simulink model "logic"  (R2023a)
settings: Solver=FixedStepAuto  StartTime=0.0  StopTime=10.0  FixedStep=1  RelTol=1e-3
libraries: simulink x1
settings Model: Creator=Dheeraj Patil  LastModifiedBy=Dheeraj Patil

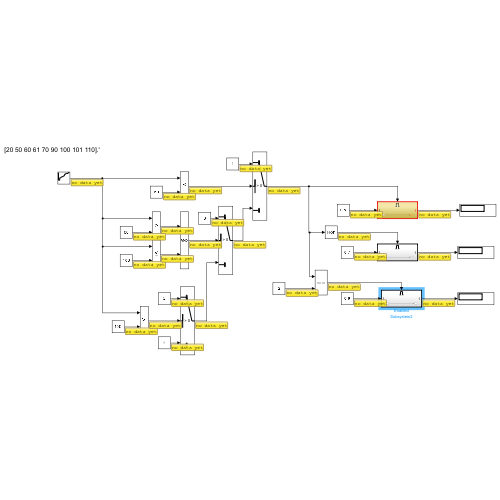
[thumbnail: Simulink's stored preview of the top-level diagram]
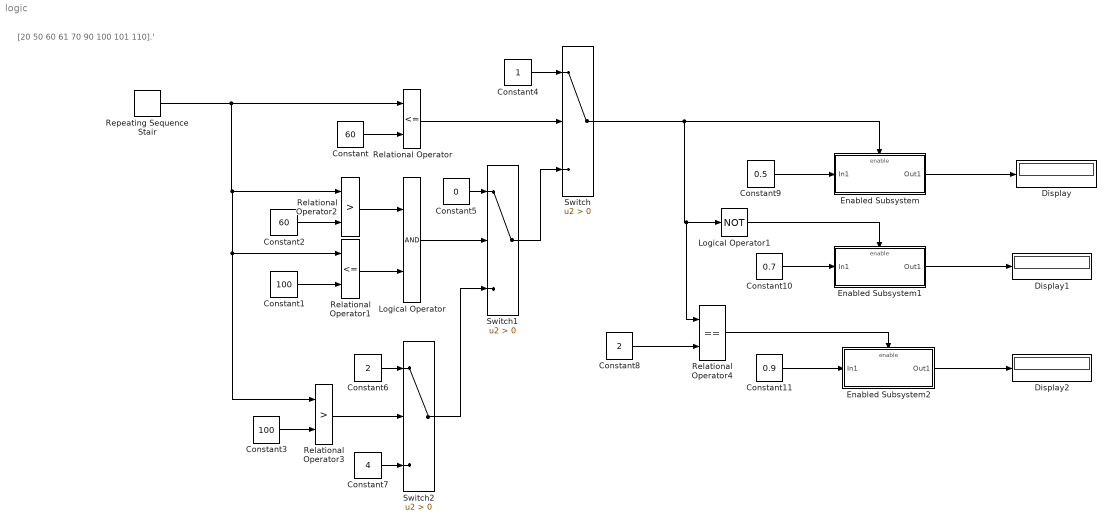
== system logic ==
  note: [20 50 60 61 70 90 100 101 110].'
  Constant : Constant  Value=60
  Constant1 : Constant  Value=100
  Constant10 : Constant  Value=0.7
  Constant11 : Constant  Value=0.9
  Constant2 : Constant  Value=60
  Constant3 : Constant  Value=100
  Constant4 : Constant
  Constant5 : Constant  Value=0
  Constant6 : Constant  Value=2
  Constant7 : Constant  Value=4
  Constant8 : Constant  Value=2
  Constant9 : Constant  Value=0.5
  Display : Display
  Display1 : Display
  Display2 : Display
  Enabled Subsystem : Subsystem  TreatAsAtomicUnit=on
      settings: LibrarySourceBlock=|
      | hdlsllib/Ports &
      | Subsystems/Enabled
      | Subsystem
  Enabled Subsystem1 : Subsystem  TreatAsAtomicUnit=on
      settings: LibrarySourceBlock=|
      | hdlsllib/Ports &
      | Subsystems/Enabled
      | Subsystem
  Enabled Subsystem2 : Subsystem  TreatAsAtomicUnit=on
      settings: LibrarySourceBlock=|
      | hdlsllib/Ports &
      | Subsystems/Enabled
      | Subsystem
  Logical Operator : Logic  AllPortsSameDT=off  OutDataTypeStr=boolean
  Logical Operator1 : Logic  Operator=NOT  AllPortsSameDT=off  OutDataTypeStr=boolean
  Relational Operator : RelationalOperator  Operator=<=  OutDataTypeStr=boolean  RndMeth=Simplest  InputSameDT=off
  Relational Operator1 : RelationalOperator  Operator=<=  OutDataTypeStr=boolean  RndMeth=Simplest  InputSameDT=off
  Relational Operator2 : RelationalOperator  Operator=>  OutDataTypeStr=boolean  RndMeth=Simplest  InputSameDT=off
  Relational Operator3 : RelationalOperator  Operator=>  OutDataTypeStr=boolean  RndMeth=Simplest  InputSameDT=off
  Relational Operator4 : RelationalOperator  Operator===  OutDataTypeStr=boolean  RndMeth=Simplest  InputSameDT=off
  Repeating Sequence Stair : simulink/Sources/Repeating Sequence Stair  OutValues=[20 50 60 61 70 90 100 101 110].'  tsamp=-1  OutMin=[]  OutMax=[]  OutDataTypeStr=double  OutputDataTypeScalingMode=double  OutDataType=fixdt(0,8)  ConRadixGroup=Best Precision: Vector-wise  OutScaling=2^-12
  Switch : Switch  Criteria=u2 > Threshold  SaturateOnIntegerOverflow=off  InputSameDT=off
  Switch1 : Switch  Criteria=u2 > Threshold  SaturateOnIntegerOverflow=off  InputSameDT=off
  Switch2 : Switch  Criteria=u2 > Threshold  SaturateOnIntegerOverflow=off  InputSameDT=off
  wires:
  Relational Operator/1 -> Switch/2
  Constant/1 -> Relational Operator/2
  Switch1/1 -> Switch/3
  Constant1/1 -> Relational Operator1/2
  Logical Operator/1 -> Switch1/2
  Relational Operator1/1 -> Logical Operator/2
  Relational Operator2/1 -> Logical Operator/1
  Constant2/1 -> Relational Operator2/2
  Repeating Sequence Stair/1 -> Relational Operator1/1, Relational Operator3/1, Relational Operator2/1, Relational Operator/1
  Switch2/1 -> Switch1/3
  Relational Operator3/1 -> Switch2/2
  Constant3/1 -> Relational Operator3/2
  Constant4/1 -> Switch/1
  Constant5/1 -> Switch1/1
  Constant6/1 -> Switch2/1
  Constant7/1 -> Switch2/3
  Switch/1 -> Relational Operator4/1, Logical Operator1/1, Enabled Subsystem/Enable
  Logical Operator1/1 -> Enabled Subsystem1/Enable
  Constant8/1 -> Relational Operator4/2
  Relational Operator4/1 -> Enabled Subsystem2/Enable
  Enabled Subsystem/1(Out1) -> Display/1
  Constant9/1 -> Enabled Subsystem/1(In1)
  Constant10/1 -> Enabled Subsystem1/1(In1)
  Enabled Subsystem1/1(Out1) -> Display1/1
  Constant11/1 -> Enabled Subsystem2/1(In1)
  Enabled Subsystem2/1(Out1) -> Display2/1

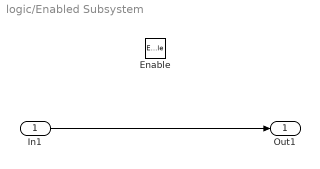
== system logic/Enabled Subsystem ==
  In1 : Inport
  Enable : EnablePort
  Out1 : Outport  OutputWhenDisabled=reset  InitialOutput=0
  wires:
  In1/1 -> Out1/1

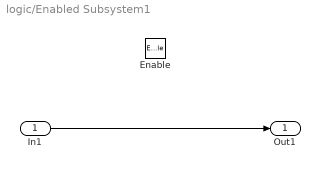
== system logic/Enabled Subsystem1 ==
  In1 : Inport
  Enable : EnablePort
  Out1 : Outport  OutputWhenDisabled=reset  InitialOutput=0
  wires:
  In1/1 -> Out1/1

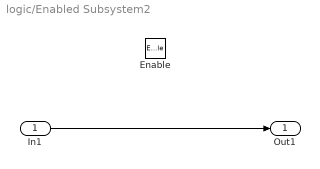
== system logic/Enabled Subsystem2 ==
  In1 : Inport
  Enable : EnablePort
  Out1 : Outport  OutputWhenDisabled=reset  InitialOutput=0
  wires:
  In1/1 -> Out1/1
